simulink model "ctrl_TAPM"  (R2015a)
settings: Solver=ode3  StartTime=0.0  StopTime=inf  FixedStep=0.01  RelTol=1e-3
undefined symbols (not defined in the file): C, D, eps_c, epsilon, hd, hd2, I_s, k_cc, K_omega, K_q1f, K_q1r, K_q2f, K_q2r, K_q3f, K_q3r, K_q4f, K_q4r, K_q5f, K_q5r, K_q6f, K_q6r, K_T1f, K_T1r, K_T2f, K_T2r, K_T3f, K_T3r, K_T4f, K_T4r, K_T5f, K_T5r, K_T6f, K_T6r, Kp, Max_Acceleration, Max_rotation, Max_thrust, Min_thrust, n_c, n_max, p_cc, pwm_thr1_backward, pwm_thr1_forward, pwm_thr2_backward, pwm_thr2_forward, pwm_thr3_backward, pwm_thr3_forward, pwm_thr4_backward, pwm_thr4_forward, pwm_thr5_backward, pwm_thr5_forward, pwm_thr6_backward, pwm_thr6_forward, Q_f0, Q_max, r_cc, Rho, Thruster
libraries: marine_gnc x10, dspstat3 x8, simulink x6, simulink_extras x3
(part 7 of 7)

== matlab function ctrl_TAPM/Thruster control /Thruster 2/Thruster control/Core controller/Core controller: Torque,Power and Combined Torque//Power ==
  data: Qcq output; Qcp output; k_cc input; p_cc input; r_cc input; n input; Qcc output; K_t0 input; K_q0 input; D input; Tr input; rho input; eps_c input; K_t0r input; K_q0r input
function [Qcq,Qcp,Qcc]= CoreControl(k_cc,p_cc,r_cc,n,K_t0,K_q0,D,Tr,rho,eps_c,K_t0r,K_q0r)
%#codegen

lambda_c = 0.5+0.5*tanh(eps_c*n/5);
K_TC = K_t0*lambda_c+(1-lambda_c)*K_t0r;
K_QC = K_q0*lambda_c+(1-lambda_c)*K_q0r;
Qcq = (K_QC/K_TC)*D*Tr;
if n == 0
    Qcp = 0;
else
Qcp = sign(Tr)*K_QC*(abs(Tr)^(3/2))/(sqrt(rho)*D*K_TC^(3/2)*abs(n));
end
alpha_c = exp(-k_cc*abs(p_cc*n)^r_cc);

Qcc = alpha_c*Qcq + (1-alpha_c)*Qcp;

== matlab function ctrl_TAPM/Thruster control /Thruster 2/Thruster control/MATLAB Function ==
  data: Td input; n_d output; K_t0 input; K_t0r input; rho input; D input; eps_c input; n_c input; n_r input; T_r output
function [n_d,T_r]  = ReferenceGenerator(Td,K_t0,K_t0r,rho,D,eps_c,n_c,n_r)
%#codegen


n_d = sign(Td)*sqrt((abs(Td))/(rho*D^4*K_t0));

lambda_c = 0.5+0.5*tanh(eps_c*n_d/5); % Smooth switching between positive and negative thrust
K_TC = K_t0*lambda_c+(1-lambda_c)*K_t0r;

T_r = sign(n_r)*K_TC*rho*D^4*n_r^2;

== matlab function ctrl_TAPM/Thruster control /Thruster 2/Thruster control/Supervisor ==
  data: control input; input input; n input; u output
function u = fcn(control,input,n)
u = 1;
if control == 1
if input == 1
    u = 1;
elseif input == 2
    u = 2;
elseif input == 3 && n > 0 || input == 3 && n < 0
    u = 3;
elseif input == 4 || input == 3 && n == 0
    u = 4;
else 
    u = 5;
end
end

if control == 2
if input == 1
    u = 1;
elseif input == 2
    u = 2;
elseif input == 3 && n > 0 || input == 3 && n < 0
    u = 3;
elseif input == 4 || input == 3 && n == 0
    u = 4;
else 
    u = 5;
end
end

if control == 3
if input == 1
    u = 1;
elseif input == 2
    u = 2;
elseif input == 3 && n > 0 || input == 3 && n < 0
    u = 3;
elseif input == 4 || input == 3 && n == 0
    u = 4;
else 
    u = 5;
end
end

if control == 4
if input == 1
    u = 1;
elseif input == 2
    u = 2;
elseif input == 3 && n > 0 || input == 3 && n < 0
    u = 3;
elseif input == 4 || input == 3 && n == 0
    u = 4;
else 
    u = 5;
end
end

if control == 5
if input == 1
    u = 1;
elseif input == 2
    u = 2;
elseif input == 3 && n > 0 || input == 3 && n < 0
    u = 3;
elseif input == 4 || input == 3 && n == 0
    u = 4;
else 
    u = 5;
end
end

== matlab function ctrl_TAPM/Thruster control /Thrust and Shaft speed mapped to PWM/MATLAB Function4 ==
  data: Tc_in1 input; signal input; Tc_out output; Tc_in2 input
function Tc_out = fcn(Tc_in1,signal,Tc_in2)
%#codegen

if signal >= 0
    Tc_out = Tc_in1;
else %signal < 0
    Tc_out = Tc_in2;
end

== matlab function ctrl_TAPM/Thruster control /Thruster 3/Propeller Hydrodynamics/Actual Force and Torque ==
  data: Ta output; n input; Qa output; Kq input; Kt input; Ktr input; Kqr input; Rho input; D input; eps_c input; env input
function [Ta,Qa]= ActualForces(n,Kq,Kt,Ktr,Kqr,Rho,D,eps_c,env)
%#codegen
lambda_c = 0.5+0.5*tanh(eps_c*n/5); % Smooth switching between positive and negative thrust. 5 makes switch happen between -5 and 5
K_TC = Kt*lambda_c+(1-lambda_c)*Ktr;
K_QC = Kq*lambda_c+(1-lambda_c)*Kqr;

Ta = sign(n)*K_TC*Rho*(D^4)*n^2-env;
Qa = sign(n)*K_QC*Rho*(D^5)*n^2-env;

== matlab function ctrl_TAPM/Input/MATLAB Function3 ==
  data: fzp output; fzp_in input
function fzp = fcn(fzp_in)
%#codegen

fzp = [fzp_in(1) fzp_in(2)]';

== matlab function ctrl_TAPM/Thruster control /Thrust and Shaft speed mapped to PWM/MATLAB Function5 ==
  data: Tc_in1 input; signal input; Tc_out output; Tc_in2 input
function Tc_out = fcn(Tc_in1,signal,Tc_in2)
%#codegen

if signal >= 0
    Tc_out = Tc_in1;
else %signal < 0
    Tc_out = Tc_in2;
end

== matlab function ctrl_TAPM/Thruster control /Thruster 3/Thruster control/Core controller/Core controller: Torque,Power and Combined Torque//Power ==
  data: Qcq output; Qcp output; k_cc input; p_cc input; r_cc input; n input; Qcc output; K_t0 input; K_q0 input; D input; Tr input; rho input; eps_c input; K_t0r input; K_q0r input
function [Qcq,Qcp,Qcc]= CoreControl(k_cc,p_cc,r_cc,n,K_t0,K_q0,D,Tr,rho,eps_c,K_t0r,K_q0r)
%#codegen

lambda_c = 0.5+0.5*tanh(eps_c*n/5);
K_TC = K_t0*lambda_c+(1-lambda_c)*K_t0r;
K_QC = K_q0*lambda_c+(1-lambda_c)*K_q0r;
Qcq = (K_QC/K_TC)*D*Tr;
if n == 0
    Qcp = 0;
else
Qcp = sign(Tr)*K_QC*(abs(Tr)^(3/2))/(sqrt(rho)*D*K_TC^(3/2)*abs(n));
end
alpha_c = exp(-k_cc*abs(p_cc*n)^r_cc);

Qcc = alpha_c*Qcq + (1-alpha_c)*Qcp;

== matlab function ctrl_TAPM/Thruster control /Thruster 3/Thruster control/MATLAB Function ==
  data: Td input; n_d output; K_t0 input; K_t0r input; rho input; D input; eps_c input; n_c input; n_r input; T_r output
function [n_d,T_r]  = ReferenceGenerator(Td,K_t0,K_t0r,rho,D,eps_c,n_c,n_r)
%#codegen


n_d = sign(Td)*sqrt((abs(Td))/(rho*D^4*K_t0));

lambda_c = 0.5+0.5*tanh(eps_c*n_d/5); % Smooth switching between positive and negative thrust
K_TC = K_t0*lambda_c+(1-lambda_c)*K_t0r;

T_r = sign(n_r)*K_TC*rho*D^4*n_r^2;

== matlab function ctrl_TAPM/Thruster control /Thrust and Shaft speed mapped to PWM/MATLAB Function ==
  data: input input; output output; control input; speedcontrol input
function output = fcn(input,control,speedcontrol)
%#codegen
if control == 1
output = [input(1) speedcontrol(1) input(3) speedcontrol(2) input(5) speedcontrol(3) input(7) speedcontrol(4) input(9) speedcontrol(5) input(11) speedcontrol(6)]';
%     output = [input(1) input(2) input(3) input(4) input(5) input(6) input(7) input(8) input(9) input(10) input(11) input(12)]';

else
    output = [input(1) input(2) input(3) input(4) input(5) input(6) input(7) input(8) input(9) input(10) input(11) input(12)]';

end

== matlab function ctrl_TAPM/Thruster control /Thrust and Shaft speed mapped to PWM/MATLAB Function6 ==
  data: Tc_in1 input; signal input; Tc_out output; Tc_in2 input
function Tc_out = fcn(Tc_in1,signal,Tc_in2)
%#codegen

if signal >= 0
    Tc_out = Tc_in1;
else %signal < 0
    Tc_out = Tc_in2;
end

== matlab function ctrl_TAPM/Input/MATLAB Function ==
  data: K_p output; K_p1 input
function K_p = fcn(K_p1)
%#codegen

K_p = diag(K_p1);

== matlab function ctrl_TAPM/Input/MATLAB Function1 ==
  data: K_i output; K_i1 input
function K_i = fcn(K_i1)
%#codegen

K_i = diag(K_i1);

== matlab function ctrl_TAPM/Thruster control /Thruster 3/Thruster control/Supervisor ==
  data: control input; input input; n input; u output
function u = fcn(control,input,n)
u = 1;
if control == 1
if input == 1
    u = 1;
elseif input == 2
    u = 2;
elseif input == 3 && n > 0 || input == 3 && n < 0
    u = 3;
elseif input == 4 || input == 3 && n == 0
    u = 4;
else 
    u = 5;
end
end

if control == 2
if input == 1
    u = 1;
elseif input == 2
    u = 2;
elseif input == 3 && n > 0 || input == 3 && n < 0
    u = 3;
elseif input == 4 || input == 3 && n == 0
    u = 4;
else 
    u = 5;
end
end

if control == 3
if input == 1
    u = 1;
elseif input == 2
    u = 2;
elseif input == 3 && n > 0 || input == 3 && n < 0
    u = 3;
elseif input == 4 || input == 3 && n == 0
    u = 4;
else 
    u = 5;
end
end

if control == 4
if input == 1
    u = 1;
elseif input == 2
    u = 2;
elseif input == 3 && n > 0 || input == 3 && n < 0
    u = 3;
elseif input == 4 || input == 3 && n == 0
    u = 4;
else 
    u = 5;
end
end

if control == 5
if input == 1
    u = 1;
elseif input == 2
    u = 2;
elseif input == 3 && n > 0 || input == 3 && n < 0
    u = 3;
elseif input == 4 || input == 3 && n == 0
    u = 4;
else 
    u = 5;
end
end

== matlab function ctrl_TAPM/Input/MATLAB Function2 ==
  data: K_d output; K_d1 input
function K_d = fcn(K_d1)
%#codegen

K_d = diag(K_d1);

== matlab function ctrl_TAPM/Thruster control /Thruster 4/Propeller Hydrodynamics/Actual Force and Torque ==
  data: Ta output; n input; Qa output; Kq input; Kt input; Ktr input; Kqr input; Rho input; D input; eps_c input; env input
function [Ta,Qa]= ActualForces(n,Kq,Kt,Ktr,Kqr,Rho,D,eps_c,env)
%#codegen
lambda_c = 0.5+0.5*tanh(eps_c*n/5); % Smooth switching between positive and negative thrust. 5 makes switch happen between -5 and 5
K_TC = Kt*lambda_c+(1-lambda_c)*Ktr;
K_QC = Kq*lambda_c+(1-lambda_c)*Kqr;

Ta = sign(n)*K_TC*Rho*(D^4)*n^2-env;
Qa = sign(n)*K_QC*Rho*(D^5)*n^2-env;

== matlab function ctrl_TAPM/Thruster control /Thruster 4/Thruster control/Core controller/Core controller: Torque,Power and Combined Torque//Power ==
  data: Qcq output; Qcp output; k_cc input; p_cc input; r_cc input; n input; Qcc output; K_t0 input; K_q0 input; D input; Tr input; rho input; eps_c input; K_t0r input; K_q0r input
function [Qcq,Qcp,Qcc]= CoreControl(k_cc,p_cc,r_cc,n,K_t0,K_q0,D,Tr,rho,eps_c,K_t0r,K_q0r)
%#codegen

lambda_c = 0.5+0.5*tanh(eps_c*n/5);
K_TC = K_t0*lambda_c+(1-lambda_c)*K_t0r;
K_QC = K_q0*lambda_c+(1-lambda_c)*K_q0r;
Qcq = (K_QC/K_TC)*D*Tr;
if n == 0
    Qcp = 0;
else
Qcp = sign(Tr)*K_QC*(abs(Tr)^(3/2))/(sqrt(rho)*D*K_TC^(3/2)*abs(n));
end
alpha_c = exp(-k_cc*abs(p_cc*n)^r_cc);

Qcc = alpha_c*Qcq + (1-alpha_c)*Qcp;

== matlab function ctrl_TAPM/Thruster control /Thruster 4/Thruster control/MATLAB Function ==
  data: Td input; n_d output; K_t0 input; K_t0r input; rho input; D input; eps_c input; n_c input; n_r input; T_r output
function [n_d,T_r]  = ReferenceGenerator(Td,K_t0,K_t0r,rho,D,eps_c,n_c,n_r)
%#codegen


n_d = sign(Td)*sqrt((abs(Td))/(rho*D^4*K_t0));

lambda_c = 0.5+0.5*tanh(eps_c*n_d/5); % Smooth switching between positive and negative thrust
K_TC = K_t0*lambda_c+(1-lambda_c)*K_t0r;

T_r = sign(n_r)*K_TC*rho*D^4*n_r^2;

== matlab function ctrl_TAPM/Thruster control /Thruster 4/Thruster control/Supervisor ==
  data: control input; input input; n input; u output
function u = fcn(control,input,n)
u = 1;
if control == 1
if input == 1
    u = 1;
elseif input == 2
    u = 2;
elseif input == 3 && n > 0 || input == 3 && n < 0
    u = 3;
elseif input == 4 || input == 3 && n == 0
    u = 4;
else 
    u = 5;
end
end

if control == 2
if input == 1
    u = 1;
elseif input == 2
    u = 2;
elseif input == 3 && n > 0 || input == 3 && n < 0
    u = 3;
elseif input == 4 || input == 3 && n == 0
    u = 4;
else 
    u = 5;
end
end

if control == 3
if input == 1
    u = 1;
elseif input == 2
    u = 2;
elseif input == 3 && n > 0 || input == 3 && n < 0
    u = 3;
elseif input == 4 || input == 3 && n == 0
    u = 4;
else 
    u = 5;
end
end

if control == 4
if input == 1
    u = 1;
elseif input == 2
    u = 2;
elseif input == 3 && n > 0 || input == 3 && n < 0
    u = 3;
elseif input == 4 || input == 3 && n == 0
    u = 4;
else 
    u = 5;
end
end

if control == 5
if input == 1
    u = 1;
elseif input == 2
    u = 2;
elseif input == 3 && n > 0 || input == 3 && n < 0
    u = 3;
elseif input == 4 || input == 3 && n == 0
    u = 4;
else 
    u = 5;
end
end

== matlab function ctrl_TAPM/TAPM Controller w_observer/PID/MATLAB Function ==
  data: reset output; timer input; rmax input; y output; eta input
function [reset,y] = fcn(timer,rmax,eta)
persistent controller res tmp

if (isempty(controller))
     controller = 1;
     tmp = 0;
end

res = 0;

pos = sqrt(eta(1)^2+eta(2)^2);

    if pos > rmax && controller ~=2
        controller = 2;
        res = 1;
    elseif pos < 0.9*rmax && timer > 40 && controller ~= 1 && tmp > 190
        controller = 1;
        res = 1;
    end
    
    if pos > rmax 
        res = 1;
        tmp = 0;
    else
        tmp = tmp + 0.01;
    end

    y = controller;
    reset = res;
    
end

== matlab function ctrl_TAPM/Thruster control /Thruster 5/Propeller Hydrodynamics/Actual Force and Torque ==
  data: Ta output; n input; Qa output; Kq input; Kt input; Ktr input; Kqr input; Rho input; D input; eps_c input; env input
function [Ta,Qa]= ActualForces(n,Kq,Kt,Ktr,Kqr,Rho,D,eps_c,env)
%#codegen
lambda_c = 0.5+0.5*tanh(eps_c*n/5); % Smooth switching between positive and negative thrust. 5 makes switch happen between -5 and 5
K_TC = Kt*lambda_c+(1-lambda_c)*Ktr;
K_QC = Kq*lambda_c+(1-lambda_c)*Kqr;

Ta = sign(n)*K_TC*Rho*(D^4)*n^2-env;
Qa = sign(n)*K_QC*Rho*(D^5)*n^2-env;

== matlab function ctrl_TAPM/Thruster control /Thruster 5/Thruster control/Core controller/Core controller: Torque,Power and Combined Torque//Power ==
  data: Qcq output; Qcp output; k_cc input; p_cc input; r_cc input; n input; Qcc output; K_t0 input; K_q0 input; D input; Tr input; rho input; eps_c input; K_t0r input; K_q0r input
function [Qcq,Qcp,Qcc]= CoreControl(k_cc,p_cc,r_cc,n,K_t0,K_q0,D,Tr,rho,eps_c,K_t0r,K_q0r)
%#codegen

lambda_c = 0.5+0.5*tanh(eps_c*n/5);
K_TC = K_t0*lambda_c+(1-lambda_c)*K_t0r;
K_QC = K_q0*lambda_c+(1-lambda_c)*K_q0r;
Qcq = (K_QC/K_TC)*D*Tr;
if n == 0
    Qcp = 0;
else
Qcp = sign(Tr)*K_QC*(abs(Tr)^(3/2))/(sqrt(rho)*D*K_TC^(3/2)*abs(n));
end
alpha_c = exp(-k_cc*abs(p_cc*n)^r_cc);

Qcc = alpha_c*Qcq + (1-alpha_c)*Qcp;

== matlab function ctrl_TAPM/Thruster control /Thruster 5/Thruster control/MATLAB Function ==
  data: Td input; n_d output; K_t0 input; K_t0r input; rho input; D input; eps_c input; n_c input; n_r input; T_r output
function [n_d,T_r]  = ReferenceGenerator(Td,K_t0,K_t0r,rho,D,eps_c,n_c,n_r)
%#codegen


n_d = sign(Td)*sqrt((abs(Td))/(rho*D^4*K_t0));

lambda_c = 0.5+0.5*tanh(eps_c*n_d/5); % Smooth switching between positive and negative thrust
K_TC = K_t0*lambda_c+(1-lambda_c)*K_t0r;

T_r = sign(n_r)*K_TC*rho*D^4*n_r^2;

== matlab function ctrl_TAPM/Thruster control /Thruster 5/Thruster control/Supervisor ==
  data: control input; input input; n input; u output
function u = fcn(control,input,n)
u = 1;
if control == 1
if input == 1
    u = 1;
elseif input == 2
    u = 2;
elseif input == 3 && n > 0 || input == 3 && n < 0
    u = 3;
elseif input == 4 || input == 3 && n == 0
    u = 4;
else 
    u = 5;
end
end

if control == 2
if input == 1
    u = 1;
elseif input == 2
    u = 2;
elseif input == 3 && n > 0 || input == 3 && n < 0
    u = 3;
elseif input == 4 || input == 3 && n == 0
    u = 4;
else 
    u = 5;
end
end

if control == 3
if input == 1
    u = 1;
elseif input == 2
    u = 2;
elseif input == 3 && n > 0 || input == 3 && n < 0
    u = 3;
elseif input == 4 || input == 3 && n == 0
    u = 4;
else 
    u = 5;
end
end

if control == 4
if input == 1
    u = 1;
elseif input == 2
    u = 2;
elseif input == 3 && n > 0 || input == 3 && n < 0
    u = 3;
elseif input == 4 || input == 3 && n == 0
    u = 4;
else 
    u = 5;
end
end

if control == 5
if input == 1
    u = 1;
elseif input == 2
    u = 2;
elseif input == 3 && n > 0 || input == 3 && n < 0
    u = 3;
elseif input == 4 || input == 3 && n == 0
    u = 4;
else 
    u = 5;
end
end

== matlab function ctrl_TAPM/Input/MATLAB Function4 ==
  data: K_p output; K_p1 input
function K_p = fcn(K_p1)
%#codegen

K_p = diag(K_p1);

== matlab function ctrl_TAPM/Thruster control /Thruster 6/Propeller Hydrodynamics/Actual Force and Torque ==
  data: Ta output; n input; Qa output; Kq input; Kt input; Ktr input; Kqr input; Rho input; D input; eps_c input; env input
function [Ta,Qa]= ActualForces(n,Kq,Kt,Ktr,Kqr,Rho,D,eps_c,env)
%#codegen
lambda_c = 0.5+0.5*tanh(eps_c*n/5); % Smooth switching between positive and negative thrust. 5 makes switch happen between -5 and 5
K_TC = Kt*lambda_c+(1-lambda_c)*Ktr;
K_QC = Kq*lambda_c+(1-lambda_c)*Kqr;

Ta = sign(n)*K_TC*Rho*(D^4)*n^2-env;
Qa = sign(n)*K_QC*Rho*(D^5)*n^2-env;

== matlab function ctrl_TAPM/Thruster control /Thruster 6/Thruster control/Core controller/Core controller: Torque,Power and Combined Torque//Power ==
  data: Qcq output; Qcp output; k_cc input; p_cc input; r_cc input; n input; Qcc output; K_t0 input; K_q0 input; D input; Tr input; rho input; eps_c input; K_t0r input; K_q0r input
function [Qcq,Qcp,Qcc]= CoreControl(k_cc,p_cc,r_cc,n,K_t0,K_q0,D,Tr,rho,eps_c,K_t0r,K_q0r)
%#codegen

lambda_c = 0.5+0.5*tanh(eps_c*n/5);
K_TC = K_t0*lambda_c+(1-lambda_c)*K_t0r;
K_QC = K_q0*lambda_c+(1-lambda_c)*K_q0r;
Qcq = (K_QC/K_TC)*D*Tr;
if n == 0
    Qcp = 0;
else
Qcp = sign(Tr)*K_QC*(abs(Tr)^(3/2))/(sqrt(rho)*D*K_TC^(3/2)*abs(n));
end
alpha_c = exp(-k_cc*abs(p_cc*n)^r_cc);

Qcc = alpha_c*Qcq + (1-alpha_c)*Qcp;

== matlab function ctrl_TAPM/Thruster control /Thruster 6/Thruster control/MATLAB Function ==
  data: Td input; n_d output; K_t0 input; K_t0r input; rho input; D input; eps_c input; n_c input; n_r input; T_r output
function [n_d,T_r]  = ReferenceGenerator(Td,K_t0,K_t0r,rho,D,eps_c,n_c,n_r)
%#codegen


n_d = sign(Td)*sqrt((abs(Td))/(rho*D^4*K_t0));

lambda_c = 0.5+0.5*tanh(eps_c*n_d/27); % Smooth switching between positive and negative thrust
K_TC = K_t0*lambda_c+(1-lambda_c)*K_t0r;

T_r = sign(n_r)*K_TC*rho*D^4*n_r^2;

== matlab function ctrl_TAPM/Thruster control /Thruster 6/Thruster control/Supervisor ==
  data: control input; input input; n input; u output
function u = fcn(control,input,n)
u = 1;
if control == 1
if input == 1
    u = 1;
elseif input == 2
    u = 2;
elseif input == 3 && n > 0 || input == 3 && n < 0
    u = 3;
elseif input == 4 || input == 3 && n == 0
    u = 4;
else 
    u = 5;
end
end

if control == 2
if input == 1
    u = 1;
elseif input == 2
    u = 2;
elseif input == 3 && n > 0 || input == 3 && n < 0
    u = 3;
elseif input == 4 || input == 3 && n == 0
    u = 4;
else 
    u = 5;
end
end

if control == 3
if input == 1
    u = 1;
elseif input == 2
    u = 2;
elseif input == 3 && n > 0 || input == 3 && n < 0
    u = 3;
elseif input == 4 || input == 3 && n == 0
    u = 4;
else 
    u = 5;
end
end

if control == 4
if input == 1
    u = 1;
elseif input == 2
    u = 2;
elseif input == 3 && n > 0 || input == 3 && n < 0
    u = 3;
elseif input == 4 || input == 3 && n == 0
    u = 4;
else 
    u = 5;
end
end

if control == 5
if input == 1
    u = 1;
elseif input == 2
    u = 2;
elseif input == 3 && n > 0 || input == 3 && n < 0
    u = 3;
elseif input == 4 || input == 3 && n == 0
    u = 4;
else 
    u = 5;
end
end

== matlab function ctrl_TAPM/Input/MATLAB Function5 ==
  data: K_i output; K_i1 input
function K_i = fcn(K_i1)
%#codegen

K_i = diag(K_i1);

== matlab function ctrl_TAPM/Input/MATLAB Function6 ==
  data: K_d output; K_d1 input
function K_d = fcn(K_d1)
%#codegen

K_d = diag(K_d1);

== matlab function ctrl_TAPM/IMU/Wild point cleaner/MATLAB Function ==
  data: V_hist input; Y input; V_hist1 output; Y_prev input; Y_filtered output
function [V_hist1, Y_filtered] = outlier_clean(V_hist, Y, Y_prev)

%Calculate median and standard deviation of 5 previous voltage
med_V = median(V_hist);
mad_V = median(abs(V_hist-med_V));
std_V = 1.4826*mad_V;

if abs(Y(7)-med_V)>2*std_V  %Outlier
    Y_filtered = Y_prev;
    V_hist1 = V_hist;
else
    Y_filtered = Y;
    V_hist1 = [V_hist(2:5); Y(7)];
end

== matlab function ctrl_TAPM/TAPM Controller w_observer/LQR/MATLAB Function ==
  data: reset output; timer input; rmax input; y output; eta input
function [reset,y] = fcn(timer,rmax,eta)
persistent controller res tmp

if (isempty(controller))
     controller = 1;
     tmp = 0;
end

res = 0;

pos = sqrt(eta(1)^2+eta(2)^2);

    if pos > rmax && controller ~=2
        controller = 2;
        res = 1;
    elseif pos < 0.9*rmax && timer > 40 && controller ~= 1 && tmp > 190
        controller = 1;
        res = 1;
    end
    
    if pos > rmax 
        res = 1;
        tmp = 0;
    else
        tmp = tmp + 0.01;
    end

    y = controller;
    reset = res;
    
end

== matlab function ctrl_TAPM/TAPM Controller w_observer/LQR/MATLAB Function1 ==
  data: r input; tau output; x_hat input; bias input
function tau = fcn(r,x_hat,bias)

K =[    0.0072          0         0             7.33        0           0
         0              0.0072    -0.0011         0         7.355    0.0195
         0               0          0.72         0           0.0115    10.6236];

P =[    0.0072         0         0
         0    0.0072  -0.0011
         0   0    0.72];

psi = x_hat(3);     

R  = [cos(psi) -sin(psi) 0;
        sin(psi) cos(psi) 0
        0           0      1];     

tau = P*r-K*x_hat;

end
